simulink model "DRPLDM"  (R2019a)
settings: Solver=FixedStepAuto  StartTime=0.0  StopTime=TimeVector(end)  FixedStep=Tsim  RelTol=1e-3  EnableMultiTasking=on
values from neighbouring files (symbols this model uses):
  Ad = 0.9048    [RunModel.m]
  B1DELTT = [1 100 130]    [RunModel.m]
  B1ERPM = [0 20000 23000]    [RunModel.m]
  B1NOOILT = [300 450 573]    [RunModel.m]
  B2DELTT = [1 40 120]    [RunModel.m]
  B2ERPM = [0 20000 23000]    [RunModel.m]
  B2NOOILT = [300 400 530]    [RunModel.m]
  B3DELTT = [1 50 110]    [RunModel.m]
  B3ERPM = [0 20000 23000]    [RunModel.m]
  B3NOOILT = [300 410 540]    [RunModel.m]
  Bd = 0.1903    [RunModel.m]
  BoosterVec = [hex2dec('55'), hex2dec('AA') hex2dec('FF')]    [RunModel.m]
  Cd = -0.5    [RunModel.m]
  Dd = 0    [RunModel.m]
  DigKeys = bin2dec('0101011')    [RunModel.m]
  EngUnits = 1    [RunModel.m]
  ExComTime = ExComTime + DeltaTimeEnd    [RunModel.m]
  ExComVec = [hex2dec('AA'), hex2dec('00'), hex2dec('CC')]    [RunModel.m]
  ExtFPModel = 0    [RunModel.m]
  FlightStart = 0    [RunModel.m]
  HILMode = 1    [RunModel.m]
  LeverMode = 1    [RunModel.m]
  Mode = 0    [RunModel.m]
  Mwm = 0.35    [RunModel.m]
  OPRPMMax = 4500    [RunModel.m]
  SensFaultStartTime = SensFaultStartTime + DeltaTimeEnd    [RunModel.m]
  SensFaultStopTime = SensFaultStopTime + DeltaTimeEnd    [RunModel.m]
  SysFaultStartTime = SysFaultStartTime + DeltaTimeEnd    [RunModel.m]
  SysFaultStopTime = SysFaultStopTime + DeltaTimeEnd    [RunModel.m]
  TBear1Init = 0    [RunModel.m]
  TBear2Init = 0    [RunModel.m]
  TBear3Init = 0    [RunModel.m]
  Tsim = 0.001 * TICK    [RunModel.m]
  WhichCont = 2    [RunModel.m]
  WhichEngine = 1    [RunModel.m]
undefined symbols (not defined in the file or in its folder): BiasSens, BoosterLStatusTime, BoosterRStatusTime
libraries: Lib_Solve_ModelSource_TMATS x5, simulink x5
(part 2 of 2)

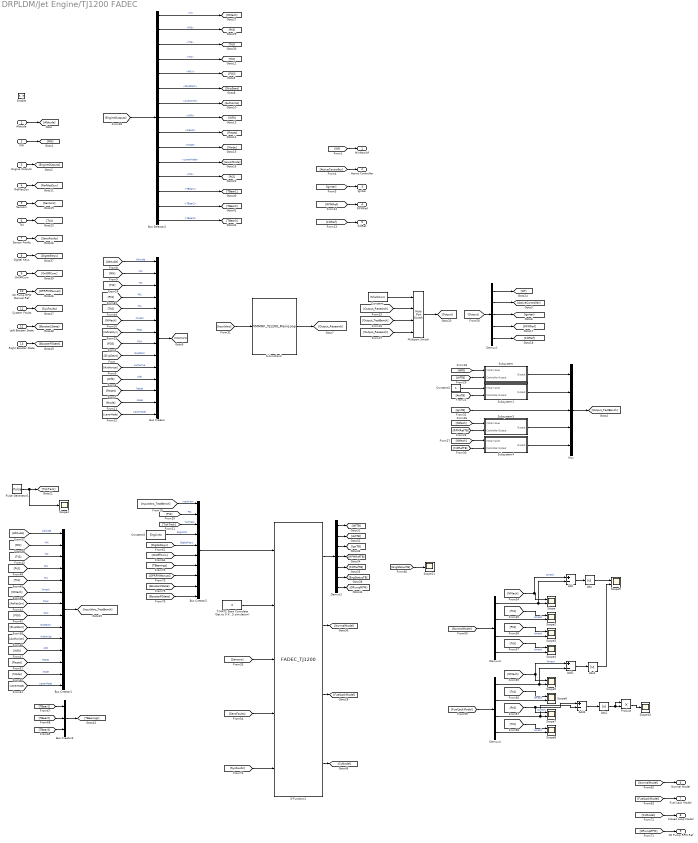
== system DRPLDM/Jet Engine/TJ1200 FADEC ==
  Altitude : Inport
  MN : Inport  Port=2
  Engine Outputs : Inport  Port=3
  RefVecDyn : Inport  Port=4
  Sensors : Inport  Port=5
  Tt4 : Inport  Port=6
  Sensor Faults : Inport  Port=7
  Digital Keys : Inport  Port=8
  OnOffCom : Inport  Port=9
  Oil Pump RPM Manual Ref : Inport  Port=10
  System Faults : Inport  Port=11
  Left Booster State : Inport  Port=12
  Right Booster State : Inport  Port=13
  Enable : EnablePort
  Abs : Abs
  Abs1 : Abs
  Abs2 : Abs
  Add : Sum  Inputs=+-
  Add1 : Sum  Inputs=+-
  Add2 : Sum  Inputs=+-
  Bus Creator : BusCreator  Inputs=14
  Bus Creator1 : BusCreator  Inputs=14
  Bus Creator2 : BusCreator  Inputs=10
  Bus Creator3 : BusCreator  Inputs=3
  Bus Selector2 : BusSelector  OutputSignals=N,Pt3,Tt5,Tt2,POil,SkipStart,Authorize,Wf0,Reset,Mode,LeverMode,Pt2,TBear1,TBear2,TBear3
  Constant : Constant  Value=WhichCont
  Constant2 : Constant
  Constant3 : Constant  Value=EngUnits
  Demux1 : Demux  Outputs=5
  Demux2 : Demux  Outputs=7
  Demux3 : Demux
  Demux4 : Demux
  Multiport Switch : MultiPortSwitch
  Mux : Mux  Inputs=5
  Product : Product
  Pulse Generator1 : DiscretePulseGenerator  PulseType=Time based  Period=2 * 0.001 * 200  PulseWidth=50
  S-Function1 : S-Function  FunctionName=FADEC_TJ1200  SFunctionDeploymentMode=off  EnableBusSupport=off
  S-Function2 : S-Function  FunctionName=PIMMRF_TJ1200_MainLoop  SFunctionDeploymentMode=off  EnableBusSupport=off
  Scope{,2..9} (9 alike) : Scope  NumInputPorts=2
  Scope1 : Scope
  Scope10 : Scope
  Scope11 : Scope
  Subsystem : Subsystem
  Subsystem1 : Subsystem
  Subsystem3 : Subsystem
  Subsystem4 : Subsystem
  T-MATS Start Complete (Set to 0 if not T-MATS simulation) : Constant  Value=0
  MinMaxWf : Outport
  Active Controller : Outport  Port=2  InitialOutput=0
  Igniter : Outport  Port=3  InitialOutput=0
  RPMRef : Outport  Port=4  InitialOutput=0
  FiltRef : Outport  Port=5  InitialOutput=0
  Normal Model : Outport  Port=6
  Fuel Lack Model : Outport  Port=7
  Closed Loop Model : Outport  Port=8
  Oil Pump RPM Ref : Outport  Port=9
  wires:
  Bus Selector2/4 -> [Tt2]  "<Tt2>"
  Altitude/1 -> [Altitude]
  MN/1 -> [MN]
  Engine Outputs/1 -> [EngineOutputs]
  RefVecDyn/1 -> [RefVecDyn]
  [EngineOutputs] -> Bus Selector2/1
  Bus Selector2/1 -> [NMech]  "<N>"
  Bus Selector2/2 -> [Pt3]  "<Pt3>"
  Bus Selector2/3 -> [Tt5]  "<Tt5>"
  [Wf] -> MinMaxWf/1
  [ActiveController] -> Active Controller/1
  [Altitude] -> Bus Creator/1  "Altitude"
  [MN] -> Bus Creator/2  "MN"
  Bus Creator/1 -> [InputVars]
  [InputVars] -> S-Function2/1
  S-Function2/1 -> [Output_Research]
  [Output] -> Demux1/1
  Demux1/2 -> [ActiveController]
  [Tt2] -> Bus Creator/3  "Tt2"
  [Pt3] -> Bus Creator/4  "Pt3"
  [Tt5] -> Bus Creator/5  "Tt4"
  [NMech] -> Bus Creator/6  "Nmech"
  [RefVecDyn] -> Bus Creator/7  "FNpc"
  Bus Selector2/5 -> [POil]  "<POil>"
  [POil] -> Bus Creator/8  "POil"
  Demux1/3 -> [Igniter]
  [Igniter] -> Igniter/1
  Bus Selector2/6 -> [SkipStart]  "<SkipStart>"
  [SkipStart] -> Bus Creator/9  "SkipStart"
  Bus Selector2/7 -> [Authorize]  "<Authorize>"
  Bus Selector2/8 -> [Wf0]  "<Wf0>"
  [Authorize] -> Bus Creator/10  "Authorize"
  [Wf0] -> Bus Creator/11  "Wf0"
  Bus Selector2/9 -> [Reset]  "<Reset>"
  [Reset] -> Bus Creator/12  "Reset"
  Bus Selector2/10 -> [Mode]  "<Mode>"
  Bus Selector2/11 -> [LeverMode]  "<LeverMode>"
  [Mode] -> Bus Creator/13  "Mode"
  [LeverMode] -> Bus Creator/14  "LeverMode"
  Demux1/4 -> [RPMRef]
  Demux1/5 -> [FiltRef]
  [FiltRef] -> FiltRef/1
  [RPMRef] -> RPMRef/1
  [Output_TestBench] -> Multiport Switch/3
  Multiport Switch/1 -> [Output]
  [Output_Research] -> Multiport Switch/4
  [Output_Research] -> Multiport Switch/2
  Constant/1 -> Multiport Switch/1
  Pulse Generator1/1 -> Scope1/1, [TickTack]
  [InputVars_TestBench] -> Bus Creator2/1  "InputVars"
  Bus Creator2/1 -> S-Function1/1
  [TickTack] -> Bus Creator2/3  "TickTack"
  [Pt2] -> Bus Creator2/2  "Pt2"
  Bus Selector2/12 -> [Pt2]  "<Pt2>"
  T-MATS Start Complete (Set to 0 if not T-MATS simulation)/1 -> S-Function1/2
  S-Function1/1 -> Demux2/1
  Demux1/1 -> [Wf]
  Subsystem/1(Output) -> Mux/1
  [Wf0] -> Subsystem/1(Initial Value)
  Constant2/1 -> Subsystem1/1(Initial Value)
  Subsystem1/1(Output) -> Mux/2
  [NMech] -> Subsystem3/1(Initial Value)
  Subsystem3/1(Output) -> Mux/4
  Subsystem4/1(Output) -> Mux/5
  [NMech] -> Subsystem4/1(Initial Value)
  [WfTB] -> Subsystem/2(Controller Output)
  Demux2/1 -> [WfTB]
  Demux2/2 -> [ActTB]
  Demux2/3 -> [IgnTB]
  Demux2/4 -> [RPMRefTB]
  Demux2/5 -> [FiltRefTB]
  [ActTB] -> Subsystem1/2(Controller Output)
  [RPMRefTB] -> Subsystem3/2(Controller Output)
  [FiltRefTB] -> Subsystem4/2(Controller Output)
  Mux/1 -> [Output_TestBench]
  [IgnTB] -> Mux/3
  Constant3/1 -> Bus Creator2/4  "EngUnits"
  Sensors/1 -> [Sensors]
  [Sensors] -> S-Function1/3
  S-Function1/2 -> [NormalModel]
  [NMech] -> Add/1, Scope/1  "Nmech"
  Demux3/1 -> Add/2, Scope/2
  Demux3/2 -> Scope2/2
  Demux3/3 -> Scope3/2
  Demux3/4 -> Scope4/2
  [Tt4] -> Scope2/1  "Nmech"
  [Pt3] -> Scope3/1  "Nmech"
  [Tt5] -> Scope4/1  "Nmech"
  Tt4/1 -> [Tt4]
  [LeverMode] -> Bus Creator1/14  "LeverMode"
  [Mode] -> Bus Creator1/13  "Mode"
  [Reset] -> Bus Creator1/12  "Reset"
  [Wf0] -> Bus Creator1/11  "Wf0"
  [Authorize] -> Bus Creator1/10  "Authorize"
  [SkipStart] -> Bus Creator1/9  "SkipStart"
  [POil] -> Bus Creator1/8  "POil"
  [RefVecDyn] -> Bus Creator1/7  "FNpc"
  [NMech] -> Bus Creator1/6  "Nmech"
  [Tt4] -> Bus Creator1/5  "Tt4"
  [Pt3] -> Bus Creator1/4  "Pt3"
  [Tt2] -> Bus Creator1/3  "Tt2"
  Bus Creator1/1 -> [InputVars_TestBench]
  [MN] -> Bus Creator1/2  "MN"
  [Altitude] -> Bus Creator1/1  "Altitude"
  Sensor Faults/1 -> [SensFaults]
  [SensFaults] -> S-Function1/4
  [Tt2] -> Scope8/1  "Nmech"
  [Pt3] -> Add2/1, Scope7/1  "Nmech"
  [Tt4] -> Scope6/1  "Nmech"
  Demux4/4 -> Scope8/2
  Demux4/3 -> Add2/2, Scope7/2
  Demux4/2 -> Scope6/2
  Demux4/1 -> Add1/2, Scope5/2
  [NMech] -> Add1/1, Scope5/1  "Nmech"
  [FuelLackModel] -> Demux4/1
  S-Function1/3 -> [FuelLackModel]
  [NormalModel] -> Demux3/1
  Add/1 -> Abs/1
  Abs/1 -> Scope9/1
  Add1/1 -> Abs1/1
  Abs1/1 -> Scope9/2
  Add2/1 -> Abs2/1
  Abs2/1 -> Product/1, Product/2
  Product/1 -> Scope10/1
  Digital Keys/1 -> [DigitalKeys]
  [DigitalKeys] -> Bus Creator2/5  "DigitalKeys"
  [NormalModel] -> Normal Model/1
  [FuelLackModel] -> Fuel Lack Model/1
  Demux2/6 -> [EngStatusTB]
  OnOffCom/1 -> [OnOffCom]
  [OnOffCom] -> Bus Creator2/6
  [EngStatusTB] -> Scope11/1
  Bus Selector2/13 -> [TBear1]  "<TBear1>"
  Bus Selector2/14 -> [TBear2]  "<TBear2>"
  Bus Selector2/15 -> [TBear3]  "<TBear3>"
  [TBear1] -> Bus Creator3/1
  [TBear2] -> Bus Creator3/2
  [TBear3] -> Bus Creator3/3
  Bus Creator3/1 -> [TBearings]
  [TBearings] -> Bus Creator2/7
  Demux2/7 -> [OPumpRPM]
  [OPumpRPM] -> Oil Pump RPM Ref/1
  S-Function1/4 -> [CLModel]
  [CLModel] -> Closed Loop Model/1
  [OPRPMManual] -> Bus Creator2/8
  Oil Pump RPM Manual Ref/1 -> [OPRPMManual]
  [SysFaults] -> S-Function1/5
  System Faults/1 -> [SysFaults]
  Right Booster State/1 -> [BoosterRState]
  Left Booster State/1 -> [BoosterLState]
  [BoosterLState] -> Bus Creator2/9
  [BoosterRState] -> Bus Creator2/10

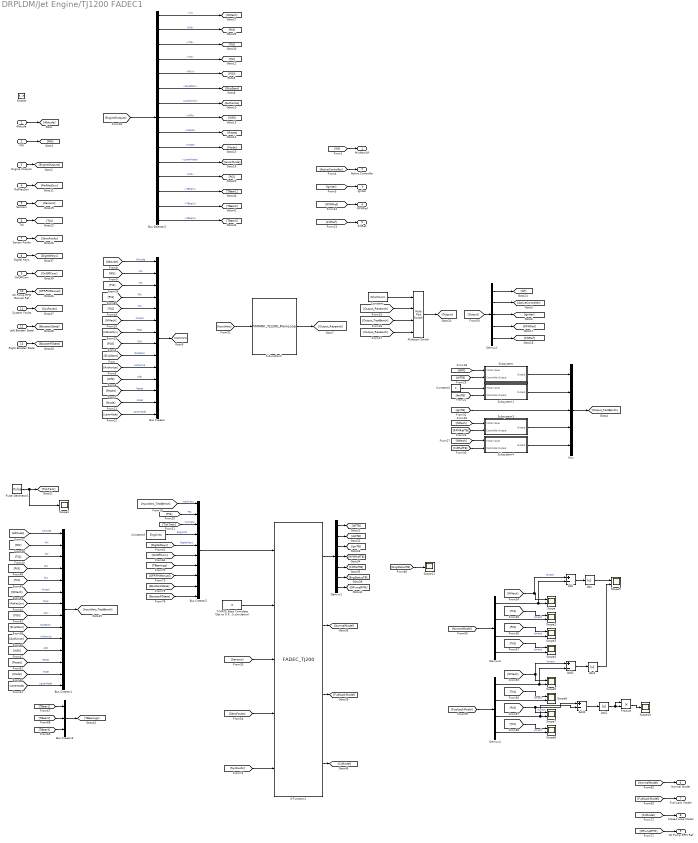
== system DRPLDM/Jet Engine/TJ1200 FADEC1 ==
  Altitude : Inport
  MN : Inport  Port=2
  Engine Outputs : Inport  Port=3
  RefVecDyn : Inport  Port=4
  Sensors : Inport  Port=5
  Tt4 : Inport  Port=6
  Sensor Faults : Inport  Port=7
  Digital Keys : Inport  Port=8
  OnOffCom : Inport  Port=9
  Oil Pump RPM Manual Ref : Inport  Port=10
  System Faults : Inport  Port=11
  Left Booster State : Inport  Port=12
  Right Booster State : Inport  Port=13
  Enable : EnablePort
  Abs : Abs
  Abs1 : Abs
  Abs2 : Abs
  Add : Sum  Inputs=+-
  Add1 : Sum  Inputs=+-
  Add2 : Sum  Inputs=+-
  Bus Creator : BusCreator  Inputs=14
  Bus Creator1 : BusCreator  Inputs=14
  Bus Creator2 : BusCreator  Inputs=10
  Bus Creator3 : BusCreator  Inputs=3
  Bus Selector2 : BusSelector  OutputSignals=N,Pt3,Tt5,Tt2,POil,SkipStart,Authorize,Wf0,Reset,Mode,LeverMode,Pt2,TBear1,TBear2,TBear3
  Constant : Constant  Value=WhichCont
  Constant2 : Constant
  Constant3 : Constant  Value=EngUnits
  Demux1 : Demux  Outputs=5
  Demux2 : Demux  Outputs=7
  Demux3 : Demux
  Demux4 : Demux
  Multiport Switch : MultiPortSwitch
  Mux : Mux  Inputs=5
  Product : Product
  Pulse Generator1 : DiscretePulseGenerator  PulseType=Time based  Period=2 * 0.001 * 200  PulseWidth=50
  S-Function1 : S-Function  FunctionName=FADEC_TJ200  SFunctionDeploymentMode=off  EnableBusSupport=off
  S-Function2 : S-Function  FunctionName=PIMMRF_TJ1200_MainLoop  SFunctionDeploymentMode=off  EnableBusSupport=off
  Scope{,2..9} (9 alike) : Scope  NumInputPorts=2
  Scope1 : Scope
  Scope10 : Scope
  Scope11 : Scope
  Subsystem : Subsystem
  Subsystem1 : Subsystem
  Subsystem3 : Subsystem
  Subsystem4 : Subsystem
  T-MATS Start Complete (Set to 0 if not T-MATS simulation) : Constant  Value=0
  MinMaxWf : Outport
  Active Controller : Outport  Port=2  InitialOutput=0
  Igniter : Outport  Port=3  InitialOutput=0
  RPMRef : Outport  Port=4  InitialOutput=0
  FiltRef : Outport  Port=5  InitialOutput=0
  Normal Model : Outport  Port=6
  Fuel Lack Model : Outport  Port=7
  Closed Loop Model : Outport  Port=8
  Oil Pump RPM Ref : Outport  Port=9
  wires:
  [BoosterRState] -> Bus Creator2/10
  [BoosterLState] -> Bus Creator2/9
  Left Booster State/1 -> [BoosterLState]
  Right Booster State/1 -> [BoosterRState]
  System Faults/1 -> [SysFaults]
  [SysFaults] -> S-Function1/5
  Oil Pump RPM Manual Ref/1 -> [OPRPMManual]
  [OPRPMManual] -> Bus Creator2/8
  [CLModel] -> Closed Loop Model/1
  S-Function1/4 -> [CLModel]
  [OPumpRPM] -> Oil Pump RPM Ref/1
  Demux2/7 -> [OPumpRPM]
  [TBearings] -> Bus Creator2/7
  Bus Creator3/1 -> [TBearings]
  [TBear3] -> Bus Creator3/3
  [TBear2] -> Bus Creator3/2
  [TBear1] -> Bus Creator3/1
  Bus Selector2/15 -> [TBear3]  "<TBear3>"
  Bus Selector2/14 -> [TBear2]  "<TBear2>"
  Bus Selector2/13 -> [TBear1]  "<TBear1>"
  [EngStatusTB] -> Scope11/1
  [OnOffCom] -> Bus Creator2/6
  OnOffCom/1 -> [OnOffCom]
  Demux2/6 -> [EngStatusTB]
  [FuelLackModel] -> Fuel Lack Model/1
  [NormalModel] -> Normal Model/1
  [DigitalKeys] -> Bus Creator2/5  "DigitalKeys"
  Digital Keys/1 -> [DigitalKeys]
  Product/1 -> Scope10/1
  Abs2/1 -> Product/2, Product/1
  Add2/1 -> Abs2/1
  Abs1/1 -> Scope9/2
  Add1/1 -> Abs1/1
  Abs/1 -> Scope9/1
  Add/1 -> Abs/1
  [NormalModel] -> Demux3/1
  S-Function1/3 -> [FuelLackModel]
  [FuelLackModel] -> Demux4/1
  [NMech] -> Scope5/1, Add1/1  "Nmech"
  Demux4/1 -> Scope5/2, Add1/2
  Demux4/2 -> Scope6/2
  Demux4/3 -> Scope7/2, Add2/2
  Demux4/4 -> Scope8/2
  [Tt4] -> Scope6/1  "Nmech"
  [Pt3] -> Scope7/1, Add2/1  "Nmech"
  [Tt2] -> Scope8/1  "Nmech"
  [SensFaults] -> S-Function1/4
  Sensor Faults/1 -> [SensFaults]
  [Altitude] -> Bus Creator1/1  "Altitude"
  [MN] -> Bus Creator1/2  "MN"
  Bus Creator1/1 -> [InputVars_TestBench]
  [Tt2] -> Bus Creator1/3  "Tt2"
  [Pt3] -> Bus Creator1/4  "Pt3"
  [Tt4] -> Bus Creator1/5  "Tt4"
  [NMech] -> Bus Creator1/6  "Nmech"
  [RefVecDyn] -> Bus Creator1/7  "FNpc"
  [POil] -> Bus Creator1/8  "POil"
  [SkipStart] -> Bus Creator1/9  "SkipStart"
  [Authorize] -> Bus Creator1/10  "Authorize"
  [Wf0] -> Bus Creator1/11  "Wf0"
  [Reset] -> Bus Creator1/12  "Reset"
  [Mode] -> Bus Creator1/13  "Mode"
  [LeverMode] -> Bus Creator1/14  "LeverMode"
  Tt4/1 -> [Tt4]
  [Tt5] -> Scope4/1  "Nmech"
  [Pt3] -> Scope3/1  "Nmech"
  [Tt4] -> Scope2/1  "Nmech"
  Demux3/4 -> Scope4/2
  Demux3/3 -> Scope3/2
  Demux3/2 -> Scope2/2
  Demux3/1 -> Scope/2, Add/2
  [NMech] -> Scope/1, Add/1  "Nmech"
  S-Function1/2 -> [NormalModel]
  [Sensors] -> S-Function1/3
  Sensors/1 -> [Sensors]
  Constant3/1 -> Bus Creator2/4  "EngUnits"
  [IgnTB] -> Mux/3
  Mux/1 -> [Output_TestBench]
  [FiltRefTB] -> Subsystem4/2(Controller Output)
  [RPMRefTB] -> Subsystem3/2(Controller Output)
  [ActTB] -> Subsystem1/2(Controller Output)
  Demux2/5 -> [FiltRefTB]
  Demux2/4 -> [RPMRefTB]
  Demux2/3 -> [IgnTB]
  Demux2/2 -> [ActTB]
  Demux2/1 -> [WfTB]
  [WfTB] -> Subsystem/2(Controller Output)
  [NMech] -> Subsystem4/1(Initial Value)
  Subsystem4/1(Output) -> Mux/5
  Subsystem3/1(Output) -> Mux/4
  [NMech] -> Subsystem3/1(Initial Value)
  Subsystem1/1(Output) -> Mux/2
  Constant2/1 -> Subsystem1/1(Initial Value)
  [Wf0] -> Subsystem/1(Initial Value)
  Subsystem/1(Output) -> Mux/1
  Demux1/1 -> [Wf]
  S-Function1/1 -> Demux2/1
  T-MATS Start Complete (Set to 0 if not T-MATS simulation)/1 -> S-Function1/2
  Bus Selector2/12 -> [Pt2]  "<Pt2>"
  [Pt2] -> Bus Creator2/2  "Pt2"
  [TickTack] -> Bus Creator2/3  "TickTack"
  Bus Creator2/1 -> S-Function1/1
  [InputVars_TestBench] -> Bus Creator2/1  "InputVars"
  Pulse Generator1/1 -> [TickTack], Scope1/1
  Constant/1 -> Multiport Switch/1
  [Output_Research] -> Multiport Switch/2
  [Output_Research] -> Multiport Switch/4
  Multiport Switch/1 -> [Output]
  [Output_TestBench] -> Multiport Switch/3
  [RPMRef] -> RPMRef/1
  [FiltRef] -> FiltRef/1
  Demux1/5 -> [FiltRef]
  Demux1/4 -> [RPMRef]
  [LeverMode] -> Bus Creator/14  "LeverMode"
  [Mode] -> Bus Creator/13  "Mode"
  Bus Selector2/11 -> [LeverMode]  "<LeverMode>"
  Bus Selector2/10 -> [Mode]  "<Mode>"
  [Reset] -> Bus Creator/12  "Reset"
  Bus Selector2/9 -> [Reset]  "<Reset>"
  [Wf0] -> Bus Creator/11  "Wf0"
  [Authorize] -> Bus Creator/10  "Authorize"
  Bus Selector2/8 -> [Wf0]  "<Wf0>"
  Bus Selector2/7 -> [Authorize]  "<Authorize>"
  [SkipStart] -> Bus Creator/9  "SkipStart"
  Bus Selector2/6 -> [SkipStart]  "<SkipStart>"
  [Igniter] -> Igniter/1
  Demux1/3 -> [Igniter]
  [POil] -> Bus Creator/8  "POil"
  Bus Selector2/5 -> [POil]  "<POil>"
  [RefVecDyn] -> Bus Creator/7  "FNpc"
  [NMech] -> Bus Creator/6  "Nmech"
  [Tt5] -> Bus Creator/5  "Tt4"
  [Pt3] -> Bus Creator/4  "Pt3"
  [Tt2] -> Bus Creator/3  "Tt2"
  Demux1/2 -> [ActiveController]
  [Output] -> Demux1/1
  S-Function2/1 -> [Output_Research]
  [InputVars] -> S-Function2/1
  Bus Creator/1 -> [InputVars]
  [MN] -> Bus Creator/2  "MN"
  [Altitude] -> Bus Creator/1  "Altitude"
  [ActiveController] -> Active Controller/1
  [Wf] -> MinMaxWf/1
  Bus Selector2/3 -> [Tt5]  "<Tt5>"
  Bus Selector2/2 -> [Pt3]  "<Pt3>"
  Bus Selector2/1 -> [NMech]  "<N>"
  [EngineOutputs] -> Bus Selector2/1
  RefVecDyn/1 -> [RefVecDyn]
  Engine Outputs/1 -> [EngineOutputs]
  MN/1 -> [MN]
  Altitude/1 -> [Altitude]
  Bus Selector2/4 -> [Tt2]  "<Tt2>"

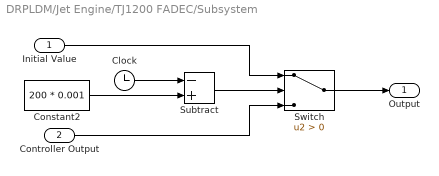
== system DRPLDM/Jet Engine/TJ1200 FADEC/Subsystem ==
  Initial Value : Inport
  Controller Output : Inport  Port=2
  Clock : Clock
  Constant2 : Constant  Value=200 * 0.001
  Subtract : Sum  Inputs=-+
  Switch : Switch  Criteria=u2 > Threshold
  Output : Outport
  wires:
  Subtract/1 -> Switch/2
  Initial Value/1 -> Switch/1
  Controller Output/1 -> Switch/3
  Switch/1 -> Output/1
  Clock/1 -> Subtract/1
  Constant2/1 -> Subtract/2

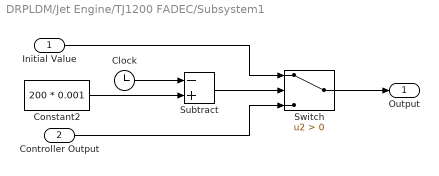
== system DRPLDM/Jet Engine/TJ1200 FADEC/Subsystem1 ==
  Initial Value : Inport
  Controller Output : Inport  Port=2
  Clock : Clock
  Constant2 : Constant  Value=200 * 0.001
  Subtract : Sum  Inputs=-+
  Switch : Switch  Criteria=u2 > Threshold
  Output : Outport
  wires:
  Constant2/1 -> Subtract/2
  Clock/1 -> Subtract/1
  Switch/1 -> Output/1
  Controller Output/1 -> Switch/3
  Initial Value/1 -> Switch/1
  Subtract/1 -> Switch/2

== system DRPLDM/Jet Engine/TJ1200 FADEC/Subsystem3 ==
  Initial Value : Inport
  Controller Output : Inport  Port=2
  Clock : Clock
  Constant2 : Constant  Value=200 * 0.001
  Subtract : Sum  Inputs=-+
  Switch : Switch  Criteria=u2 > Threshold
  Output : Outport
  wires:
  Constant2/1 -> Subtract/2
  Clock/1 -> Subtract/1
  Switch/1 -> Output/1
  Controller Output/1 -> Switch/3
  Initial Value/1 -> Switch/1
  Subtract/1 -> Switch/2

== system DRPLDM/Jet Engine/TJ1200 FADEC/Subsystem4 ==
  Initial Value : Inport
  Controller Output : Inport  Port=2
  Clock : Clock
  Constant2 : Constant  Value=200 * 0.001
  Subtract : Sum  Inputs=-+
  Switch : Switch  Criteria=u2 > Threshold
  Output : Outport
  wires:
  Subtract/1 -> Switch/2
  Initial Value/1 -> Switch/1
  Controller Output/1 -> Switch/3
  Switch/1 -> Output/1
  Clock/1 -> Subtract/1
  Constant2/1 -> Subtract/2

== system DRPLDM/Jet Engine/TJ1200 FADEC1/Subsystem ==
  Initial Value : Inport
  Controller Output : Inport  Port=2
  Clock : Clock
  Constant2 : Constant  Value=200 * 0.001
  Subtract : Sum  Inputs=-+
  Switch : Switch  Criteria=u2 > Threshold
  Output : Outport
  wires:
  Constant2/1 -> Subtract/2
  Clock/1 -> Subtract/1
  Switch/1 -> Output/1
  Controller Output/1 -> Switch/3
  Initial Value/1 -> Switch/1
  Subtract/1 -> Switch/2

== system DRPLDM/Jet Engine/TJ1200 FADEC1/Subsystem1 ==
  Initial Value : Inport
  Controller Output : Inport  Port=2
  Clock : Clock
  Constant2 : Constant  Value=200 * 0.001
  Subtract : Sum  Inputs=-+
  Switch : Switch  Criteria=u2 > Threshold
  Output : Outport
  wires:
  Subtract/1 -> Switch/2
  Initial Value/1 -> Switch/1
  Controller Output/1 -> Switch/3
  Switch/1 -> Output/1
  Clock/1 -> Subtract/1
  Constant2/1 -> Subtract/2

== system DRPLDM/Jet Engine/TJ1200 FADEC1/Subsystem3 ==
  Initial Value : Inport
  Controller Output : Inport  Port=2
  Clock : Clock
  Constant2 : Constant  Value=200 * 0.001
  Subtract : Sum  Inputs=-+
  Switch : Switch  Criteria=u2 > Threshold
  Output : Outport
  wires:
  Subtract/1 -> Switch/2
  Initial Value/1 -> Switch/1
  Controller Output/1 -> Switch/3
  Switch/1 -> Output/1
  Clock/1 -> Subtract/1
  Constant2/1 -> Subtract/2

== system DRPLDM/Jet Engine/TJ1200 FADEC1/Subsystem4 ==
  Initial Value : Inport
  Controller Output : Inport  Port=2
  Clock : Clock
  Constant2 : Constant  Value=200 * 0.001
  Subtract : Sum  Inputs=-+
  Switch : Switch  Criteria=u2 > Threshold
  Output : Outport
  wires:
  Constant2/1 -> Subtract/2
  Clock/1 -> Subtract/1
  Switch/1 -> Output/1
  Controller Output/1 -> Switch/3
  Initial Value/1 -> Switch/1
  Subtract/1 -> Switch/2

== matlab function DRPLDM/Jet Engine/MATLAB Function1 ==
  data: Time input; DigKeysOut output; StartTime input; StopTime input; DigKeysIn input; BitPosition input; TimePosition input
function DigKeysOut = fcn(Time, StartTime, StopTime, DigKeysIn, BitPosition, TimePosition)

%   bit 1 = 1 - Igniter		
% 	bit 2 = 1 - Shut_Off	 
% 	bit 3 = 0 - Scaveng		
% 	bit 4 = 1 - Oil Pump	
% 	bit 5 = 0 - AC_Drive	
% 	bit 6 = 1 - Emergency	
% 	bit 7 = 0 - Mode

%BitPosition = 6;

DigKeysOut = DigKeysIn;

for i = 1:length(BitPosition)
    
    % Reads nunber indicating position in StopTime and StartTime vectors
    TimePos = TimePosition(i);
    BitPos = BitPosition(i);
    
    if (Time < StopTime(TimePos))&&(Time > StartTime(TimePos))
        
        Bit = bitget(DigKeysIn,BitPos);
        Bit = 1 - Bit;
        DigKeysOut = bitset(DigKeysIn,BitPos,Bit);
        
%     else
%         
%         DigKeysOut = DigKeys
        
    end
    
end

== matlab function DRPLDM/Jet Engine/MATLAB Function4 ==
  data: Time input; Output output; ExComTime input; Command input
function Output = fcn(Time, ExComTime, Command)

%Position 

% 1 - Engine Start
% 2 - Nominal Engine Shut Down
% 3 - Emergency

Output = hex2dec('FF');

%Verifies which commands have been requested. Priority order:
%Emergency > Shut Down > Start
for i = 1:length(ExComTime)
    if (Time > ExComTime(i))
        
        Output = Command(i);
        
    end
end

== matlab function DRPLDM/Jet Engine/MATLAB Function2 ==
  data: Time input; Bits output; StartTime input; StopTime input; IntRep output
function [Bits,IntRep]  = fcn(Time, StartTime, StopTime)

    IntRep = 0;
    %Declares a static variable u
    persistent u;
        
    %Initiates the static variable u
    if isempty(u)
        u = zeros(1,length(StartTime)+ 1);
    end

    %Stores the bit indicating that thermocouples' fault simulation must be
    %performed by software
    %u(end) = SoftSim;
    
    %Computes the SoftSim flat in int representation
    IntRep = u(end) * 2 ^ (length(u) - 1);
    
    %Executes loop verifying if Time is between StartTime and StopTime for
    %each individual fault setting. If true, fault must be simulated
    for i = 1:length(StartTime)
%     for i = 1:(length(StartTime)-1)
        
        if (Time < StopTime(i))&&(Time > StartTime(i))
            
            u(i) = 1;
            
        else
            
            u(i) = 0;
            
        end
        
        %Adds corresponding integer decimal term
        IntRep = IntRep + u(i) * 2^(i-1);
        
    end
    
Bits = u;

== matlab function DRPLDM/Jet Engine/MATLAB Function3 ==
  data: Time input; Bits output; StartTime input; StopTime input; IntRep output
function [Bits,IntRep]  = fcn(Time, StartTime, StopTime)

    IntRep = 0;
    %Declares a static variable u
    persistent u;
        
    %Initiates the static variable u
    if isempty(u)
        u = zeros(1,length(StartTime)+ 1);
    end

    %Stores the bit indicating that thermocouples' fault simulation must be
    %performed by software
    %u(end) = SoftSim;
    
    %Computes the SoftSim flat in int representation
    IntRep = u(end) * 2 ^ (length(u) - 1);
    
    %Executes loop verifying if Time is between StartTime and StopTime for
    %each individual fault setting. If true, fault must be simulated
    for i = 1:length(StartTime)
%     for i = 1:(length(StartTime)-1)
        
        if (Time < StopTime(i))&&(Time > StartTime(i))
            
            u(i) = 1;
            
        else
            
            u(i) = 0;
            
        end
        
        %Adds corresponding integer decimal term
        IntRep = IntRep + u(i) * 2^(i-1);
        
    end
    
Bits = u;

== matlab function DRPLDM/Jet Engine/MATLAB Function5 ==
  data: Time input; Output output; ExComTime input; Command input
function Output = fcn(Time, ExComTime, Command)

%Position 

% 1 - Engine Start
% 2 - Nominal Engine Shut Down
% 3 - Emergency

Output = hex2dec('FF');

%Verifies which commands have been requested. Priority order:
%Emergency > Shut Down > Start
for i = 1:length(ExComTime)
    if (Time > ExComTime(i))
        
        Output = Command(i);
        
    end
end

== matlab function DRPLDM/Jet Engine/MATLAB Function6 ==
  data: Time input; Output output; ExComTime input; Command input
function Output = fcn(Time, ExComTime, Command)

%Position 

% 1 - Engine Start
% 2 - Nominal Engine Shut Down
% 3 - Emergency

Output = hex2dec('FF');

%Verifies which commands have been requested. Priority order:
%Emergency > Shut Down > Start
for i = 1:length(ExComTime)
    if (Time > ExComTime(i))
        
        Output = Command(i);
        
    end
end

== matlab function DRPLDM/Jet Engine/MATLAB Function7 ==
  data: SysFaultBits input; CAN0 output; Position input; CAN1 output
function [CAN0, CAN1]  = fcn(SysFaultBits, Position)
  
    CAN0 = SysFaultBits(Position(1));
    CAN1 = SysFaultBits(Position(2));
